simulink model "p1_digital_twin"  (R2024a)
settings: Solver=FixedStepDiscrete  StartTime=0.0  StopTime=10  FixedStep=Ts  RelTol=1e-3  EnableMultiTasking=on
PreLoadFcn:
  | p1_params_new
  | SteeringController
  | addpath('./sFunctions/')
  | make
InitFcn:
  | p1_params_new
  | SteeringController
  | addpath('./sFunctions/')
  | make
values from neighbouring files (symbols this model uses):
  ack = 1    [SteeringController.m]
  cpr_handwheel = 500*4    (= 2000)    [p1_params_new.m]
  cpr_steering = 1000*4    (= 4000)    [p1_params_new.m]
  hal_filter_den = [1 1*(2*pi*Ts)-1]    [SteeringController.m]    (also in p1_params_new.m = DEN_cellarray{1})
  hal_filter_num = [1*(2*pi*Ts)]    [SteeringController.m]    (also in p1_params_new.m = NUM_cellarray{1})
  n_drive = 5.6    [p1_params_new.m]
  n_handwheel = 50    [p1_params_new.m]
  n_steering = 160    [p1_params_new.m]
  sr = 7.5    [SteeringController.m]
  steering_limit = 35    [SteeringController.m]
  Ts = 0.001    [p1_params_new.m]
  wc = 10    [SteeringController.m]    (also in p1_params_new.m = p1params.input.VAccelFc*(2*Ts))
undefined symbols (not defined in the file or in its folder): DiscIntNeverNeededParam, p1params, param
libraries: simulink x7
(part 3 of 3)

== system p1_digital_twin/Driver and Controller Input/Steering Controller/HAL-9000 ==
  Trigger : Inport
  Amplitude : Constant  Value=amplitude*sr*pi/180
  Chirp Signal : Subsystem  mask(chirp){f1=startfreq, T=duration, f2=endfreq, VectorParams1D=on}
      mask prompts: f1 "Initial frequency (Hz):"; T "Target time (secs):"; f2 "Frequency at target time (Hz):"; VectorParams1D "Interpret vectors parameters as 1-D"
      mask help: Output a linear chirp signal (sine wave whose frequency varies linearly with time).
      mask init:
      | blkName = gcb;
      | t=[0:.1:5];
      | set_param([blkName '/targetTime'], 'VectorParams1D', VectorParams1D);
      | set_param([blkName '/initialFreq'], 'VectorParams1D', VectorParams1D);
      | set_param([blkName '/deltaFreq'], 'VectorParams1D', VectorParams1D);
      mask Help: The chirp signal has linearly increasing frequency with time.  This block can be used for spectral analysis of nonlinear systems.
      mask Display: plot(t,sin(t.*t))
  Constant : Constant
  Constant1 : Constant  Value=0
  Delay : Constant  Value=delay
  Digital Clock : DigitalClock  SampleTime=Ts
  Double chirp : Subsystem
  Double-step : Subsystem
      mask Display: plot([0 1 1 2 2 3 3 4 4 5],[0 0 1 1 0 0 -1 -1 0 0])
  Enable : Constant  Value=enabled
  Latch : Subsystem  TreatAsAtomicUnit=on
  Maneuver : Constant  Value=maneuver
  Multiport Switch : MultiPortSwitch  Inputs=5  SaturateOnIntegerOverflow=off  InputSameDT=off
  Product : Product  Inputs=3  SaturateOnIntegerOverflow=on  OutDataTypeStr=Inherit: Same as first input
  Product1 : Product  SaturateOnIntegerOverflow=on  OutDataTypeStr=Inherit: Same as first input
  Ramp : Subsystem
      mask Display: plot([0 3 7 10],[1 1 8 8])
  Step : Subsystem
      mask Display: plot([0 5 5 10],[1 1 8 8])
  Sum : Sum  Inputs=|++
  Switch : Switch  Criteria=u2 ~= 0  SaturateOnIntegerOverflow=off  InputSameDT=off
  Offset : Outport
  wires:
  Double chirp/1(Out1) -> Multiport Switch/6
  Double-step/1(Out) -> Multiport Switch/5
  Enable/1 -> Product1/2
  Trigger/1 -> Switch/2
  Delay/1 -> Sum/2
  Latch/1(Out1) -> Sum/1
  Chirp Signal/1(Out2) -> Multiport Switch/4
  Ramp/1(Out1) -> Multiport Switch/3
  Sum/1 -> Double chirp/1(In1), Double-step/1(Start Time), Chirp Signal/1(Start Time), Ramp/1(Start Time), Step/1(Start Time)
  Maneuver/1 -> Multiport Switch/1
  Step/1(Out) -> Multiport Switch/2
  Amplitude/1 -> Product/3
  Multiport Switch/1 -> Product/2
  Product/1 -> Offset/1
  Product1/1 -> Latch/Trigger, Product/1
  Digital Clock/1 -> Latch/1(In1)
  Switch/1 -> Product1/1
  Constant1/1 -> Switch/3
  Constant/1 -> Switch/1

== system p1_digital_twin/Vehicle Chassis Dynamics/Lateral Brush Tire Model/Sgn with deadband ==
  In : Inport
  Dead Zone : DeadZone  LowerValue=-lower_dz  UpperValue=upper_dz  ZeroCross=off
  Sign : Signum  ZeroCross=off
  Out : Outport  VectorParamsAs1DForOutWhenUnconnected=off
  wires:
  In/1 -> Dead Zone/1
  Dead Zone/1 -> Sign/1
  Sign/1 -> Out/1

== system p1_digital_twin/Vehicle Chassis Dynamics/WFT Emulation/WFT Byte Packing ==
  In1 : Inport
  Data Type Conversion2 : DataTypeConversion  OutDataTypeStr=int16  SaturateOnIntegerOverflow=off  RndMeth=Floor
  S-Function5 : S-Function  FunctionName=int16ToBytes  SFunctionDeploymentMode=off  EnableBusSupport=off
  WFT Fy unscaling : Gain  Gain=1/0.6103515625
  Out1 : Outport
  Out2 : Outport  Port=2
  wires:
  WFT Fy unscaling/1 -> Data Type Conversion2/1
  Data Type Conversion2/1 -> S-Function5/1
  In1/1 -> WFT Fy unscaling/1
  S-Function5/1 -> Out2/1, Out1/1

== system p1_digital_twin/Vehicle Chassis Dynamics/WFT Emulation/WFT Byte Packing1 ==
  In1 : Inport
  Data Type Conversion2 : DataTypeConversion  OutDataTypeStr=int16  SaturateOnIntegerOverflow=off  RndMeth=Floor
  S-Function5 : S-Function  FunctionName=int16ToBytes  SFunctionDeploymentMode=off  EnableBusSupport=off
  WFT Fy unscaling : Gain  Gain=1/0.6103515625
  Out1 : Outport
  Out2 : Outport  Port=2
  wires:
  WFT Fy unscaling/1 -> Data Type Conversion2/1
  Data Type Conversion2/1 -> S-Function5/1
  In1/1 -> WFT Fy unscaling/1
  S-Function5/1 -> Out2/1, Out1/1

== system p1_digital_twin/Vehicle Chassis Dynamics/WFT Emulation/WFT Byte Packing10 ==
  In1 : Inport
  Data Type Conversion2 : DataTypeConversion  OutDataTypeStr=int16  SaturateOnIntegerOverflow=off  RndMeth=Floor
  S-Function5 : S-Function  FunctionName=int16ToBytes  SFunctionDeploymentMode=off  EnableBusSupport=off
  WFT Fy unscaling : Gain  Gain=1/0.6103515625
  Out1 : Outport
  Out2 : Outport  Port=2
  wires:
  In1/1 -> WFT Fy unscaling/1
  Data Type Conversion2/1 -> S-Function5/1
  WFT Fy unscaling/1 -> Data Type Conversion2/1
  S-Function5/1 -> Out2/1, Out1/1

== system p1_digital_twin/Vehicle Chassis Dynamics/WFT Emulation/WFT Byte Packing11 ==
  In1 : Inport
  Data Type Conversion2 : DataTypeConversion  OutDataTypeStr=int16  SaturateOnIntegerOverflow=off  RndMeth=Floor
  S-Function5 : S-Function  FunctionName=int16ToBytes  SFunctionDeploymentMode=off  EnableBusSupport=off
  WFT Fy unscaling : Gain  Gain=1/0.6103515625
  Out1 : Outport
  Out2 : Outport  Port=2
  wires:
  In1/1 -> WFT Fy unscaling/1
  Data Type Conversion2/1 -> S-Function5/1
  WFT Fy unscaling/1 -> Data Type Conversion2/1
  S-Function5/1 -> Out2/1, Out1/1

== system p1_digital_twin/Vehicle Chassis Dynamics/WFT Emulation/WFT Byte Packing12 ==
  In1 : Inport
  Data Type Conversion2 : DataTypeConversion  OutDataTypeStr=int16  SaturateOnIntegerOverflow=off  RndMeth=Floor
  S-Function5 : S-Function  FunctionName=int16ToBytes  SFunctionDeploymentMode=off  EnableBusSupport=off
  WFT Fy unscaling : Gain  Gain=1/0.6103515625
  Out1 : Outport
  Out2 : Outport  Port=2
  wires:
  WFT Fy unscaling/1 -> Data Type Conversion2/1
  Data Type Conversion2/1 -> S-Function5/1
  In1/1 -> WFT Fy unscaling/1
  S-Function5/1 -> Out2/1, Out1/1

== system p1_digital_twin/Vehicle Chassis Dynamics/WFT Emulation/WFT Byte Packing13 ==
  In1 : Inport
  Data Type Conversion2 : DataTypeConversion  OutDataTypeStr=int16  SaturateOnIntegerOverflow=off  RndMeth=Floor
  S-Function5 : S-Function  FunctionName=int16ToBytes  SFunctionDeploymentMode=off  EnableBusSupport=off
  WFT Fy unscaling : Gain  Gain=1/0.6103515625
  Out1 : Outport
  Out2 : Outport  Port=2
  wires:
  WFT Fy unscaling/1 -> Data Type Conversion2/1
  Data Type Conversion2/1 -> S-Function5/1
  In1/1 -> WFT Fy unscaling/1
  S-Function5/1 -> Out2/1, Out1/1

== system p1_digital_twin/Vehicle Chassis Dynamics/WFT Emulation/WFT Byte Packing14 ==
  In1 : Inport
  Data Type Conversion2 : DataTypeConversion  OutDataTypeStr=int16  SaturateOnIntegerOverflow=off  RndMeth=Floor
  S-Function5 : S-Function  FunctionName=int16ToBytes  SFunctionDeploymentMode=off  EnableBusSupport=off
  WFT Fy unscaling : Gain  Gain=1/0.6103515625
  Out1 : Outport
  Out2 : Outport  Port=2
  wires:
  WFT Fy unscaling/1 -> Data Type Conversion2/1
  Data Type Conversion2/1 -> S-Function5/1
  In1/1 -> WFT Fy unscaling/1
  S-Function5/1 -> Out2/1, Out1/1

== system p1_digital_twin/Vehicle Chassis Dynamics/WFT Emulation/WFT Byte Packing15 ==
  In1 : Inport
  Data Type Conversion2 : DataTypeConversion  OutDataTypeStr=int16  SaturateOnIntegerOverflow=off  RndMeth=Floor
  S-Function5 : S-Function  FunctionName=int16ToBytes  SFunctionDeploymentMode=off  EnableBusSupport=off
  WFT Fy unscaling : Gain  Gain=1/0.6103515625
  Out1 : Outport
  Out2 : Outport  Port=2
  wires:
  WFT Fy unscaling/1 -> Data Type Conversion2/1
  Data Type Conversion2/1 -> S-Function5/1
  In1/1 -> WFT Fy unscaling/1
  S-Function5/1 -> Out2/1, Out1/1

== system p1_digital_twin/Vehicle Chassis Dynamics/WFT Emulation/WFT Byte Packing16 ==
  In1 : Inport
  Data Type Conversion2 : DataTypeConversion  OutDataTypeStr=int16  SaturateOnIntegerOverflow=off  RndMeth=Floor
  S-Function5 : S-Function  FunctionName=int16ToBytes  SFunctionDeploymentMode=off  EnableBusSupport=off
  WFT Fy unscaling : Gain  Gain=1/0.6103515625
  Out1 : Outport
  Out2 : Outport  Port=2
  wires:
  In1/1 -> WFT Fy unscaling/1
  Data Type Conversion2/1 -> S-Function5/1
  WFT Fy unscaling/1 -> Data Type Conversion2/1
  S-Function5/1 -> Out2/1, Out1/1

== system p1_digital_twin/Vehicle Chassis Dynamics/WFT Emulation/WFT Byte Packing17 ==
  In1 : Inport
  Data Type Conversion2 : DataTypeConversion  OutDataTypeStr=int16  SaturateOnIntegerOverflow=off  RndMeth=Floor
  S-Function5 : S-Function  FunctionName=int16ToBytes  SFunctionDeploymentMode=off  EnableBusSupport=off
  WFT Fy unscaling : Gain  Gain=1/0.6103515625
  Out1 : Outport
  Out2 : Outport  Port=2
  wires:
  In1/1 -> WFT Fy unscaling/1
  Data Type Conversion2/1 -> S-Function5/1
  WFT Fy unscaling/1 -> Data Type Conversion2/1
  S-Function5/1 -> Out2/1, Out1/1

== system p1_digital_twin/Vehicle Chassis Dynamics/WFT Emulation/WFT Byte Packing18 ==
  In1 : Inport
  Data Type Conversion2 : DataTypeConversion  OutDataTypeStr=int16  SaturateOnIntegerOverflow=off  RndMeth=Floor
  S-Function5 : S-Function  FunctionName=int16ToBytes  SFunctionDeploymentMode=off  EnableBusSupport=off
  WFT Fy unscaling : Gain  Gain=1/0.6103515625
  Out1 : Outport
  Out2 : Outport  Port=2
  wires:
  In1/1 -> WFT Fy unscaling/1
  Data Type Conversion2/1 -> S-Function5/1
  WFT Fy unscaling/1 -> Data Type Conversion2/1
  S-Function5/1 -> Out2/1, Out1/1

== system p1_digital_twin/Vehicle Chassis Dynamics/WFT Emulation/WFT Byte Packing19 ==
  In1 : Inport
  Data Type Conversion2 : DataTypeConversion  OutDataTypeStr=int16  SaturateOnIntegerOverflow=off  RndMeth=Floor
  S-Function5 : S-Function  FunctionName=int16ToBytes  SFunctionDeploymentMode=off  EnableBusSupport=off
  WFT Fy unscaling : Gain  Gain=1/0.6103515625
  Out1 : Outport
  Out2 : Outport  Port=2
  wires:
  WFT Fy unscaling/1 -> Data Type Conversion2/1
  Data Type Conversion2/1 -> S-Function5/1
  In1/1 -> WFT Fy unscaling/1
  S-Function5/1 -> Out2/1, Out1/1

== system p1_digital_twin/Vehicle Chassis Dynamics/WFT Emulation/WFT Byte Packing2 ==
  In1 : Inport
  Data Type Conversion2 : DataTypeConversion  OutDataTypeStr=int16  SaturateOnIntegerOverflow=off  RndMeth=Floor
  S-Function5 : S-Function  FunctionName=int16ToBytes  SFunctionDeploymentMode=off  EnableBusSupport=off
  WFT Fy unscaling : Gain  Gain=1/0.6103515625
  Out1 : Outport
  Out2 : Outport  Port=2
  wires:
  In1/1 -> WFT Fy unscaling/1
  Data Type Conversion2/1 -> S-Function5/1
  WFT Fy unscaling/1 -> Data Type Conversion2/1
  S-Function5/1 -> Out2/1, Out1/1

== system p1_digital_twin/Vehicle Chassis Dynamics/WFT Emulation/WFT Byte Packing3 ==
  In1 : Inport
  Data Type Conversion2 : DataTypeConversion  OutDataTypeStr=int16  SaturateOnIntegerOverflow=off  RndMeth=Floor
  S-Function5 : S-Function  FunctionName=int16ToBytes  SFunctionDeploymentMode=off  EnableBusSupport=off
  WFT Fy unscaling : Gain  Gain=1/0.6103515625
  Out1 : Outport
  Out2 : Outport  Port=2
  wires:
  In1/1 -> WFT Fy unscaling/1
  Data Type Conversion2/1 -> S-Function5/1
  WFT Fy unscaling/1 -> Data Type Conversion2/1
  S-Function5/1 -> Out2/1, Out1/1

== system p1_digital_twin/Vehicle Chassis Dynamics/WFT Emulation/WFT Byte Packing4 ==
  In1 : Inport
  Data Type Conversion2 : DataTypeConversion  OutDataTypeStr=int16  SaturateOnIntegerOverflow=off  RndMeth=Floor
  S-Function5 : S-Function  FunctionName=int16ToBytes  SFunctionDeploymentMode=off  EnableBusSupport=off
  WFT Fy unscaling : Gain  Gain=1/0.6103515625
  Out1 : Outport
  Out2 : Outport  Port=2
  wires:
  In1/1 -> WFT Fy unscaling/1
  Data Type Conversion2/1 -> S-Function5/1
  WFT Fy unscaling/1 -> Data Type Conversion2/1
  S-Function5/1 -> Out2/1, Out1/1

== system p1_digital_twin/Vehicle Chassis Dynamics/WFT Emulation/WFT Byte Packing5 ==
  In1 : Inport
  Data Type Conversion2 : DataTypeConversion  OutDataTypeStr=int16  SaturateOnIntegerOverflow=off  RndMeth=Floor
  S-Function5 : S-Function  FunctionName=int16ToBytes  SFunctionDeploymentMode=off  EnableBusSupport=off
  WFT Fy unscaling : Gain  Gain=1/0.6103515625
  Out1 : Outport
  Out2 : Outport  Port=2
  wires:
  In1/1 -> WFT Fy unscaling/1
  Data Type Conversion2/1 -> S-Function5/1
  WFT Fy unscaling/1 -> Data Type Conversion2/1
  S-Function5/1 -> Out2/1, Out1/1

== system p1_digital_twin/Vehicle Chassis Dynamics/WFT Emulation/WFT Byte Packing6 ==
  In1 : Inport
  Data Type Conversion2 : DataTypeConversion  OutDataTypeStr=int16  SaturateOnIntegerOverflow=off  RndMeth=Floor
  S-Function5 : S-Function  FunctionName=int16ToBytes  SFunctionDeploymentMode=off  EnableBusSupport=off
  WFT Fy unscaling : Gain  Gain=1/0.6103515625
  Out1 : Outport
  Out2 : Outport  Port=2
  wires:
  WFT Fy unscaling/1 -> Data Type Conversion2/1
  Data Type Conversion2/1 -> S-Function5/1
  In1/1 -> WFT Fy unscaling/1
  S-Function5/1 -> Out2/1, Out1/1

== system p1_digital_twin/Vehicle Chassis Dynamics/WFT Emulation/WFT Byte Packing7 ==
  In1 : Inport
  Data Type Conversion2 : DataTypeConversion  OutDataTypeStr=int16  SaturateOnIntegerOverflow=off  RndMeth=Floor
  S-Function5 : S-Function  FunctionName=int16ToBytes  SFunctionDeploymentMode=off  EnableBusSupport=off
  WFT Fy unscaling : Gain  Gain=1/0.6103515625
  Out1 : Outport
  Out2 : Outport  Port=2
  wires:
  WFT Fy unscaling/1 -> Data Type Conversion2/1
  Data Type Conversion2/1 -> S-Function5/1
  In1/1 -> WFT Fy unscaling/1
  S-Function5/1 -> Out2/1, Out1/1

== system p1_digital_twin/Vehicle Chassis Dynamics/WFT Emulation/WFT Byte Packing8 ==
  In1 : Inport
  Data Type Conversion2 : DataTypeConversion  OutDataTypeStr=int16  SaturateOnIntegerOverflow=off  RndMeth=Floor
  S-Function5 : S-Function  FunctionName=int16ToBytes  SFunctionDeploymentMode=off  EnableBusSupport=off
  WFT Fy unscaling : Gain  Gain=1/0.6103515625
  Out1 : Outport
  Out2 : Outport  Port=2
  wires:
  WFT Fy unscaling/1 -> Data Type Conversion2/1
  Data Type Conversion2/1 -> S-Function5/1
  In1/1 -> WFT Fy unscaling/1
  S-Function5/1 -> Out2/1, Out1/1

== system p1_digital_twin/Vehicle Chassis Dynamics/WFT Emulation/WFT Byte Packing9 ==
  In1 : Inport
  Data Type Conversion2 : DataTypeConversion  OutDataTypeStr=int16  SaturateOnIntegerOverflow=off  RndMeth=Floor
  S-Function5 : S-Function  FunctionName=int16ToBytes  SFunctionDeploymentMode=off  EnableBusSupport=off
  WFT Fy unscaling : Gain  Gain=1/0.6103515625
  Out1 : Outport
  Out2 : Outport  Port=2
  wires:
  In1/1 -> WFT Fy unscaling/1
  Data Type Conversion2/1 -> S-Function5/1
  WFT Fy unscaling/1 -> Data Type Conversion2/1
  S-Function5/1 -> Out2/1, Out1/1

== system p1_digital_twin/Driver and Controller Input/Steering Controller/HAL-9000/Chirp Signal ==
  note: freqSlope = deltaFreq/targetTime;
      | instantaneousFreq(t) = freqSlope*t + initialFreq;
      | intantaneousPhase(t) = integral(instFreq) = ...
      |       0.5*freqSlope*t^2 + initialFreq*t;
      | outputSignal(t) = sin(instantaneousPhase(t));
  Start Time : Inport
  Digital Clock : DigitalClock  SampleTime=Ts
  Gain : Gain  DisableCoverage=on  Gain=0.5  OutDataTypeStr=Inherit: Same as input  ParamDataTypeStr=Inherit: Same as input
  Output : Trigonometry
  Product : Product  DisableCoverage=on  Inputs=*/  InputSameDT=on  SaturateOnIntegerOverflow=on  OutDataTypeStr=Inherit: Same as first input
  Product1 : Product  DisableCoverage=on  InputSameDT=on  SaturateOnIntegerOverflow=on  OutDataTypeStr=Inherit: Same as first input
  Product2 : Product  DisableCoverage=on  InputSameDT=on  SaturateOnIntegerOverflow=on  OutDataTypeStr=Inherit: Same as first input
  Saturation : Saturate  UpperLimit=duration  LowerLimit=0
  Sum : Sum  DisableCoverage=on  Inputs=|++  InputSameDT=on  SaturateOnIntegerOverflow=on  OutDataTypeStr=Inherit: Same as first input
  Sum1 : Sum  DisableCoverage=on  Inputs=-+|  InputSameDT=on  SaturateOnIntegerOverflow=on  OutDataTypeStr=Inherit: Same as first input
  deltaFreq : Constant  DisableCoverage=on  Value=2*pi*(f2-f1)
  initialFreq : Constant  DisableCoverage=on  Value=2*pi*f1
  targetTime : Constant  DisableCoverage=on  Value=T
  Out2 : Outport
  wires:
  Sum1/1 -> Saturation/1
  Digital Clock/1 -> Sum1/2
  Start Time/1 -> Sum1/1
  deltaFreq/1 -> Product/1
  targetTime/1 -> Product/2
  Product/1 -> Gain/1
  Gain/1 -> Product1/2
  Product1/1 -> Sum/1
  initialFreq/1 -> Sum/2
  Sum/1 -> Product2/2
  Product2/1 -> Output/1
  Output/1 -> Out2/1
  Saturation/1 -> Product1/1, Product2/1

== system p1_digital_twin/Driver and Controller Input/Steering Controller/HAL-9000/Double chirp ==
  In1 : Inport
  Chirp One : Subsystem  mask(chirp){f1=startfreq, T=duration/2, f2=endfreq, VectorParams1D=on}
      mask prompts: f1 "Initial frequency (Hz):"; T "Target time (secs):"; f2 "Frequency at target time (Hz):"; VectorParams1D "Interpret vectors parameters as 1-D"
      mask help: Output a linear chirp signal (sine wave whose frequency varies linearly with time).
      mask init: same as p1_digital_twin/Driver and Controller Input/Steering Controller/HAL-9000/Chirp Signal
      mask Help: The chirp signal has linearly increasing frequency with time.  This block can be used for spectral analysis of nonlinear systems.
      mask Display: plot(t,sin(t.*t))
  Chirp Two : Subsystem  mask(chirp){f1=startfreq, T=duration/2, f2=endfreq, VectorParams1D=on}
      mask prompts: f1 "Initial frequency (Hz):"; T "Target time (secs):"; f2 "Frequency at target time (Hz):"; VectorParams1D "Interpret vectors parameters as 1-D"
      mask help: Output a linear chirp signal (sine wave whose frequency varies linearly with time).
      mask init: same as p1_digital_twin/Driver and Controller Input/Steering Controller/HAL-9000/Chirp Signal
      mask Help: The chirp signal has linearly increasing frequency with time.  This block can be used for spectral analysis of nonlinear systems.
      mask Display: plot(t,sin(t.*t))
  Digital Clock : DigitalClock  SampleTime=Ts
  Relational Operator : RelationalOperator  Operator=<=  OutDataTypeStr=float('double')  InputSameDT=off
  Sum : Sum  DisableCoverage=on  Inputs=++|  InputSameDT=on  SaturateOnIntegerOverflow=on  OutDataTypeStr=Inherit: Same as first input
  Switch : Switch  Threshold=.5  SaturateOnIntegerOverflow=off  InputSameDT=off
  initialFreq : Constant  DisableCoverage=on  Value=duration/2
  Out1 : Outport
  wires:
  Digital Clock/1 -> Relational Operator/1
  Relational Operator/1 -> Switch/2
  initialFreq/1 -> Sum/2
  Sum/1 -> Relational Operator/2, Chirp Two/1(Start Time)
  In1/1 -> Sum/1, Chirp One/1(Start Time)
  Switch/1 -> Out1/1
  Chirp Two/1(Out2) -> Switch/3
  Chirp One/1(Out2) -> Switch/1

== system p1_digital_twin/Driver and Controller Input/Steering Controller/HAL-9000/Double-step ==
  Start Time : Inport
  Data Type Conversion : DataTypeConversion  OutDataTypeStr=double  SaturateOnIntegerOverflow=off  RndMeth=Floor
  Data Type Conversion1 : DataTypeConversion  OutDataTypeStr=double  SaturateOnIntegerOverflow=off  RndMeth=Floor
  Digital Clock : DigitalClock  SampleTime=Ts
  Left Pulse : simulink/Logic and Bit Operations/Interval Test  IntervalClosedRight=off  uplimit=duration  IntervalClosedLeft=on  lowlimit=0  OutDataTypeStr=boolean
  Right Pulse : simulink/Logic and Bit Operations/Interval Test  IntervalClosedRight=off  uplimit=3*duration  IntervalClosedLeft=on  lowlimit=2*duration  OutDataTypeStr=boolean
  Sum : Sum  Inputs=+|-
  Sum1 : Sum  Inputs=+|-
  Out : Outport
  wires:
  Data Type Conversion1/1 -> Sum1/2
  Data Type Conversion/1 -> Sum1/1
  Left Pulse/1 -> Data Type Conversion/1
  Right Pulse/1 -> Data Type Conversion1/1
  Sum1/1 -> Out/1
  Sum/1 -> Right Pulse/1, Left Pulse/1
  Digital Clock/1 -> Sum/1
  Start Time/1 -> Sum/2

== system p1_digital_twin/Driver and Controller Input/Steering Controller/HAL-9000/Latch ==
  In1 : Inport
  Trigger : TriggerPort  VariantControl=(inherit)
  Out1 : Outport
  wires:
  In1/1 -> Out1/1

== system p1_digital_twin/Driver and Controller Input/Steering Controller/HAL-9000/Ramp ==
  Start Time : Inport
  Digital Clock : DigitalClock  SampleTime=Ts
  Saturation : Saturate  UpperLimit=1  LowerLimit=0
  Slope : Gain  Gain=1/duration
  Sum : Sum  DisableCoverage=on  Inputs=|+-  InputSameDT=on  SaturateOnIntegerOverflow=on  OutDataTypeStr=Inherit: Same as first input
  Out1 : Outport
  wires:
  Slope/1 -> Saturation/1
  Saturation/1 -> Out1/1
  Sum/1 -> Slope/1
  Start Time/1 -> Sum/2
  Digital Clock/1 -> Sum/1

== system p1_digital_twin/Driver and Controller Input/Steering Controller/HAL-9000/Step ==
  Start Time : Inport
  Digital Clock : DigitalClock  SampleTime=Ts
  Relational Operator : RelationalOperator  OutDataTypeStr=float('double')  InputSameDT=off
  Out : Outport
  wires:
  Start Time/1 -> Relational Operator/2
  Digital Clock/1 -> Relational Operator/1
  Relational Operator/1 -> Out/1

== system p1_digital_twin/Driver and Controller Input/Steering Controller/HAL-9000/Double chirp/Chirp One ==
  note: freqSlope = deltaFreq/targetTime;
      | instantaneousFreq(t) = freqSlope*t + initialFreq;
      | intantaneousPhase(t) = integral(instFreq) = ...
      |       0.5*freqSlope*t^2 + initialFreq*t;
      | outputSignal(t) = sin(instantaneousPhase(t));
  Start Time : Inport
  Digital Clock : DigitalClock  SampleTime=Ts
  Gain : Gain  DisableCoverage=on  Gain=0.5  OutDataTypeStr=Inherit: Same as input  ParamDataTypeStr=Inherit: Same as input
  Output : Trigonometry
  Product : Product  DisableCoverage=on  Inputs=*/  InputSameDT=on  SaturateOnIntegerOverflow=on  OutDataTypeStr=Inherit: Same as first input
  Product1 : Product  DisableCoverage=on  InputSameDT=on  SaturateOnIntegerOverflow=on  OutDataTypeStr=Inherit: Same as first input
  Product2 : Product  DisableCoverage=on  InputSameDT=on  SaturateOnIntegerOverflow=on  OutDataTypeStr=Inherit: Same as first input
  Saturation : Saturate  UpperLimit=duration/2  LowerLimit=0
  Sum : Sum  DisableCoverage=on  Inputs=|++  InputSameDT=on  SaturateOnIntegerOverflow=on  OutDataTypeStr=Inherit: Same as first input
  Sum1 : Sum  DisableCoverage=on  Inputs=-+|  InputSameDT=on  SaturateOnIntegerOverflow=on  OutDataTypeStr=Inherit: Same as first input
  deltaFreq : Constant  DisableCoverage=on  Value=2*pi*(f2-f1)
  initialFreq : Constant  DisableCoverage=on  Value=2*pi*f1
  targetTime : Constant  DisableCoverage=on  Value=T
  Out2 : Outport
  wires:
  Sum1/1 -> Saturation/1
  Digital Clock/1 -> Sum1/2
  Start Time/1 -> Sum1/1
  deltaFreq/1 -> Product/1
  targetTime/1 -> Product/2
  Product/1 -> Gain/1
  Gain/1 -> Product1/2
  Product1/1 -> Sum/1
  initialFreq/1 -> Sum/2
  Sum/1 -> Product2/2
  Product2/1 -> Output/1
  Output/1 -> Out2/1
  Saturation/1 -> Product1/1, Product2/1

== system p1_digital_twin/Driver and Controller Input/Steering Controller/HAL-9000/Double chirp/Chirp Two ==
  note: freqSlope = deltaFreq/targetTime;
      | instantaneousFreq(t) = freqSlope*t + initialFreq;
      | intantaneousPhase(t) = integral(instFreq) = ...
      |       0.5*freqSlope*t^2 + initialFreq*t;
      | outputSignal(t) = sin(instantaneousPhase(t));
  Start Time : Inport
  Digital Clock : DigitalClock  SampleTime=Ts
  Gain : Gain  DisableCoverage=on  Gain=0.5  OutDataTypeStr=Inherit: Same as input  ParamDataTypeStr=Inherit: Same as input
  Output : Trigonometry
  Product : Product  DisableCoverage=on  Inputs=*/  InputSameDT=on  SaturateOnIntegerOverflow=on  OutDataTypeStr=Inherit: Same as first input
  Product1 : Product  DisableCoverage=on  InputSameDT=on  SaturateOnIntegerOverflow=on  OutDataTypeStr=Inherit: Same as first input
  Product2 : Product  DisableCoverage=on  InputSameDT=on  SaturateOnIntegerOverflow=on  OutDataTypeStr=Inherit: Same as first input
  Saturation : Saturate  UpperLimit=duration/2  LowerLimit=0
  Sum : Sum  DisableCoverage=on  Inputs=|++  InputSameDT=on  SaturateOnIntegerOverflow=on  OutDataTypeStr=Inherit: Same as first input
  Sum1 : Sum  DisableCoverage=on  Inputs=-+|  InputSameDT=on  SaturateOnIntegerOverflow=on  OutDataTypeStr=Inherit: Same as first input
  deltaFreq : Constant  DisableCoverage=on  Value=2*pi*(f2-f1)
  initialFreq : Constant  DisableCoverage=on  Value=2*pi*f1
  targetTime : Constant  DisableCoverage=on  Value=T
  Out2 : Outport
  wires:
  Sum1/1 -> Saturation/1
  Digital Clock/1 -> Sum1/2
  Start Time/1 -> Sum1/1
  deltaFreq/1 -> Product/1
  targetTime/1 -> Product/2
  Product/1 -> Gain/1
  Gain/1 -> Product1/2
  Product1/1 -> Sum/1
  initialFreq/1 -> Sum/2
  Sum/1 -> Product2/2
  Product2/1 -> Output/1
  Output/1 -> Out2/1
  Saturation/1 -> Product1/1, Product2/1
